simulink model "Simulink_Model"  (R2020b)
settings: Solver=FixedStepAuto  StartTime=0.0  StopTime=12  FixedStep=1  RelTol=1e-3
values from neighbouring files (symbols this model uses):
  ConstantA = Constants{1}    [Load_config.m]
  ConstantB = Constants{2}    [Load_config.m]
  ConstantC = Constants{3}    [Load_config.m]
  ConstantD = Constants{4}    [Load_config.m]
  ConstantE = Constants{5}    [Load_config.m]
  ConstantF = Constants{6}    [Load_config.m]
  ConstantG = Constants{7}    [Load_config.m]
  ConstantH = Constants{8}    [Load_config.m]
  ConstantI = Constants{9}    [Load_config.m]
  ConstantJ = Constants{18}    [Load_config.m]
  ConstantK = Constants{19}    [Load_config.m]
  ConstantL = Constants{20}    [Load_config.m]
  ConstantM = Constants{21}    [Load_config.m]
  ConstantO = Constants{22}    [Load_config.m]
undefined symbols (not defined in the file or in its folder): A1052, A2, F2, G1052, H2, K1052
libraries: simulink x32, sldvlib x22
(part 2 of 3)

== system Simulink_Model/Subsystem/Requirement3/ComputeOutputD[0][0] ==
  OutputB[x][y] : Inport
  Compare To Constant1 : simulink/Logic and Bit Operations/Compare To Constant  relop=>=  const=0  OutDataTypeStr=boolean
  Constant : Constant  Value=0.5
  Constant1 : Constant  Value=ConstantD
  Constant2 : Constant  Value=ConstantB
  Constant3 : Constant  Value=ConstantC
  Constant4 : Constant  Value=ConstantE
  Constant5 : Constant  Value=ConstantI
  Divide : Product  Inputs=*/
  Gain : Gain  Gain=-1
  Product : Product  Inputs=3
  Product1 : Product  Inputs=3
  Product2 : Product
  Sum : Sum  Inputs=|++
  Switch2 : Switch  Criteria=u2 > Threshold
  OutputD[x][y] : Outport
  wires:
  OutputB[x][y]/1 -> Product/3
  Constant1/1 -> Product/1  "ConstantD"
  Constant2/1 -> Product/2  "ConstantB"
  Constant4/1 -> Product1/2  "ConstantE"
  Constant3/1 -> Product1/1  "ConstantC"
  Constant5/1 -> Product1/3  "ConstantI"
  Product/1 -> Sum/1, Compare To Constant1/1
  Gain/1 -> Switch2/3
  Product1/1 -> Divide/2, Product2/2
  Product2/1 -> Switch2/1, Gain/1
  Constant/1 -> Product2/1
  Divide/1 -> OutputD[x][y]/1
  Sum/1 -> Divide/1
  Compare To Constant1/1 -> Switch2/2
  Switch2/1 -> Sum/2

== system Simulink_Model/Subsystem/Requirement3/ComputeOutputD[0][1] ==
  OutputB[x][y] : Inport
  Compare To Constant1 : simulink/Logic and Bit Operations/Compare To Constant  relop=>=  const=0  OutDataTypeStr=boolean
  Constant : Constant  Value=0.5
  Constant1 : Constant  Value=ConstantD
  Constant2 : Constant  Value=ConstantB
  Constant3 : Constant  Value=ConstantC
  Constant4 : Constant  Value=ConstantE
  Constant5 : Constant  Value=ConstantI
  Divide : Product  Inputs=*/
  Gain : Gain  Gain=-1
  Product : Product  Inputs=3
  Product1 : Product  Inputs=3
  Product2 : Product
  Sum : Sum  Inputs=|++
  Switch2 : Switch  Criteria=u2 > Threshold
  OutputD[x][y] : Outport
  wires:
  OutputB[x][y]/1 -> Product/3
  Constant1/1 -> Product/1  "ConstantD"
  Constant2/1 -> Product/2  "ConstantB"
  Constant4/1 -> Product1/2  "ConstantE"
  Constant3/1 -> Product1/1  "ConstantC"
  Constant5/1 -> Product1/3  "ConstantI"
  Product/1 -> Sum/1, Compare To Constant1/1
  Gain/1 -> Switch2/3
  Product1/1 -> Divide/2, Product2/2
  Product2/1 -> Switch2/1, Gain/1
  Constant/1 -> Product2/1
  Divide/1 -> OutputD[x][y]/1
  Sum/1 -> Divide/1
  Compare To Constant1/1 -> Switch2/2
  Switch2/1 -> Sum/2

== system Simulink_Model/Subsystem/Requirement3/ComputeOutputD[1][0] ==
  OutputB[x][y] : Inport
  Compare To Constant1 : simulink/Logic and Bit Operations/Compare To Constant  relop=>=  const=0  OutDataTypeStr=boolean
  Constant : Constant  Value=0.5
  Constant1 : Constant  Value=ConstantD
  Constant2 : Constant  Value=ConstantB
  Constant3 : Constant  Value=ConstantC
  Constant4 : Constant  Value=ConstantE
  Constant5 : Constant  Value=ConstantI
  Divide : Product  Inputs=*/
  Gain : Gain  Gain=-1
  Product : Product  Inputs=3
  Product1 : Product  Inputs=3
  Product2 : Product
  Sum : Sum  Inputs=|++
  Switch2 : Switch  Criteria=u2 > Threshold
  OutputD[x][y] : Outport
  wires:
  OutputB[x][y]/1 -> Product/3
  Constant1/1 -> Product/1  "ConstantD"
  Constant2/1 -> Product/2  "ConstantB"
  Constant4/1 -> Product1/2  "ConstantE"
  Constant3/1 -> Product1/1  "ConstantC"
  Constant5/1 -> Product1/3  "ConstantI"
  Product/1 -> Sum/1, Compare To Constant1/1
  Gain/1 -> Switch2/3
  Product1/1 -> Divide/2, Product2/2
  Product2/1 -> Switch2/1, Gain/1
  Constant/1 -> Product2/1
  Divide/1 -> OutputD[x][y]/1
  Sum/1 -> Divide/1
  Compare To Constant1/1 -> Switch2/2
  Switch2/1 -> Sum/2

== system Simulink_Model/Subsystem/Requirement3/ComputeOutputD[1][1] ==
  OutputB[x][y] : Inport
  Compare To Constant1 : simulink/Logic and Bit Operations/Compare To Constant  relop=>=  const=0  OutDataTypeStr=boolean
  Constant : Constant  Value=0.5
  Constant1 : Constant  Value=ConstantD
  Constant2 : Constant  Value=ConstantB
  Constant3 : Constant  Value=ConstantC
  Constant4 : Constant  Value=ConstantE
  Constant5 : Constant  Value=ConstantI
  Divide : Product  Inputs=*/
  Gain : Gain  Gain=-1
  Product : Product  Inputs=3
  Product1 : Product  Inputs=3
  Product2 : Product
  Sum : Sum  Inputs=|++
  Switch2 : Switch  Criteria=u2 > Threshold
  OutputD[x][y] : Outport
  wires:
  OutputB[x][y]/1 -> Product/3
  Constant1/1 -> Product/1  "ConstantD"
  Constant2/1 -> Product/2  "ConstantB"
  Constant4/1 -> Product1/2  "ConstantE"
  Constant3/1 -> Product1/1  "ConstantC"
  Constant5/1 -> Product1/3  "ConstantI"
  Product/1 -> Sum/1, Compare To Constant1/1
  Gain/1 -> Switch2/3
  Product1/1 -> Divide/2, Product2/2
  Product2/1 -> Switch2/1, Gain/1
  Constant/1 -> Product2/1
  Divide/1 -> OutputD[x][y]/1
  Sum/1 -> Divide/1
  Compare To Constant1/1 -> Switch2/2
  Switch2/1 -> Sum/2

== system Simulink_Model/Subsystem/Requirement4/ComputeOutput[0][0] ==
  OutputB[x][y] : Inport
  OutputD[x][y] : Inport  Port=2
  OutputEOld[x][y] : Inport  Port=3
  OutputFOld[x][y] : Inport  Port=4
  Abs : Abs
  Abs1 : Abs
  Bias : Bias  Bias=50
  Constant : Constant  Value=0
  Constant1 : Constant  Value=0
  Constant2 : Constant  Value=100
  Constant3 : Constant  Value=0
  Constant4 : Constant  Value=ConstantI
  Constant6 : Constant  Value=ConstantC
  Delay : Delay  DelayLength=1  InitialCondition=0
  Delay1 : Delay  DelayLength=1  InitialCondition=0
  Divide : Product  Inputs=*/
  Max : MinMax  Function=max  Inputs=2
  Product : Product
  Product1 : Product
  Relational Operator : RelationalOperator  Operator===  OutDataTypeStr=boolean  RndMeth=Simplest
  Relational Operator1 : RelationalOperator  Operator=>  OutDataTypeStr=boolean  RndMeth=Simplest
  Subtract : Sum  Inputs=+-
  Switch : Switch
  Switch1 : Switch
  Switch2 : Switch
  OutputE[x][y] : Outport
  OutputF[x][y] : Outport  Port=2
  wires:
  Constant/1 -> Relational Operator/1
  OutputB[x][y]/1 -> Relational Operator/2
  Relational Operator/1 -> Switch2/2, Switch/2
  Switch/1 -> Product1/1, OutputE[x][y]/1
  OutputD[x][y]/1 -> Product/1, Switch/3
  Constant1/1 -> Switch1/3, Relational Operator1/1
  OutputFOld[x][y]/1 -> Delay1/1
  Relational Operator1/1 -> Switch1/2
  OutputEOld[x][y]/1 -> Delay/1
  Switch1/1 -> Switch/1
  Switch2/1 -> OutputF[x][y]/1
  Constant4/1 -> Product/2  "ConstantI"
  Product/1 -> Abs/1
  Abs/1 -> Bias/1
  Bias/1 -> Divide/1
  Constant2/1 -> Divide/2
  Divide/1 -> Switch2/1
  Subtract/1 -> Max/1
  Constant3/1 -> Max/2
  Constant6/1 -> Product1/2  "ConstantC"
  Product1/1 -> Abs1/1
  Abs1/1 -> Subtract/2
  Max/1 -> Switch2/3
  Delay/1 -> Switch1/1
  Delay1/1 -> Subtract/1, Relational Operator1/2

== system Simulink_Model/Subsystem/Requirement4/ComputeOutput[0][1] ==
  OutputB[x][y] : Inport
  OutputD[x][y] : Inport  Port=2
  OutputEOld[x][y] : Inport  Port=3
  OutputFOld[x][y] : Inport  Port=4
  Abs : Abs
  Abs1 : Abs
  Bias : Bias  Bias=50
  Constant : Constant  Value=0
  Constant1 : Constant  Value=0
  Constant2 : Constant  Value=100
  Constant3 : Constant  Value=0
  Constant4 : Constant  Value=ConstantI
  Constant6 : Constant  Value=ConstantC
  Delay : Delay  DelayLength=1  InitialCondition=0
  Delay1 : Delay  DelayLength=1  InitialCondition=0
  Divide : Product  Inputs=*/
  Max : MinMax  Function=max  Inputs=2
  Product : Product
  Product1 : Product
  Relational Operator : RelationalOperator  Operator===  OutDataTypeStr=boolean  RndMeth=Simplest
  Relational Operator1 : RelationalOperator  Operator=>  OutDataTypeStr=boolean  RndMeth=Simplest
  Subtract : Sum  Inputs=+-
  Switch : Switch
  Switch1 : Switch
  Switch2 : Switch
  OutputE[x][y] : Outport
  OutputF[x][y] : Outport  Port=2
  wires:
  Constant/1 -> Relational Operator/1
  OutputB[x][y]/1 -> Relational Operator/2
  Relational Operator/1 -> Switch2/2, Switch/2
  Switch/1 -> OutputE[x][y]/1
  OutputD[x][y]/1 -> Product/1, Switch/3
  Constant1/1 -> Switch1/3, Relational Operator1/1
  OutputFOld[x][y]/1 -> Delay1/1
  Relational Operator1/1 -> Switch1/2
  OutputEOld[x][y]/1 -> Delay/1
  Switch1/1 -> Switch/1, Product1/1
  Switch2/1 -> OutputF[x][y]/1
  Constant4/1 -> Product/2  "ConstantI"
  Product/1 -> Abs/1
  Abs/1 -> Bias/1
  Bias/1 -> Divide/1
  Constant2/1 -> Divide/2
  Divide/1 -> Subtract/1, Switch2/1
  Subtract/1 -> Max/1
  Constant3/1 -> Max/2
  Constant6/1 -> Product1/2  "ConstantC"
  Product1/1 -> Abs1/1
  Abs1/1 -> Subtract/2
  Max/1 -> Switch2/3
  Delay/1 -> Switch1/1
  Delay1/1 -> Relational Operator1/2

== system Simulink_Model/Subsystem/Requirement4/ComputeOutput[1][0] ==
  OutputB[x][y] : Inport
  OutputD[x][y] : Inport  Port=2
  OutputEOld[x][y] : Inport  Port=3
  OutputFOld[x][y] : Inport  Port=4
  Abs : Abs
  Abs1 : Abs
  Bias : Bias  Bias=50
  Constant : Constant  Value=0
  Constant1 : Constant  Value=0
  Constant2 : Constant  Value=100
  Constant3 : Constant  Value=0
  Constant4 : Constant  Value=ConstantI
  Constant6 : Constant  Value=ConstantC
  Delay : Delay  DelayLength=1  InitialCondition=0
  Delay1 : Delay  DelayLength=1  InitialCondition=0
  Divide : Product  Inputs=*/
  Max : MinMax  Function=max  Inputs=2
  Product : Product
  Product1 : Product
  Relational Operator : RelationalOperator  Operator===  OutDataTypeStr=boolean  RndMeth=Simplest
  Relational Operator1 : RelationalOperator  Operator=>  OutDataTypeStr=boolean  RndMeth=Simplest
  Subtract : Sum  Inputs=+-
  Switch : Switch
  Switch1 : Switch
  Switch2 : Switch
  OutputE[x][y] : Outport
  OutputF[x][y] : Outport  Port=2
  wires:
  Constant/1 -> Relational Operator/1
  OutputB[x][y]/1 -> Relational Operator/2
  Relational Operator/1 -> Switch2/2, Switch/2
  Switch/1 -> OutputE[x][y]/1
  OutputD[x][y]/1 -> Product/1, Switch/3
  Constant1/1 -> Switch1/3, Relational Operator1/1
  OutputFOld[x][y]/1 -> Delay1/1
  Relational Operator1/1 -> Switch1/2
  OutputEOld[x][y]/1 -> Delay/1
  Switch1/1 -> Switch/1, Product1/1
  Switch2/1 -> OutputF[x][y]/1
  Constant4/1 -> Product/2  "ConstantI"
  Product/1 -> Abs/1
  Abs/1 -> Bias/1
  Bias/1 -> Divide/1
  Constant2/1 -> Divide/2
  Divide/1 -> Subtract/1, Switch2/1
  Subtract/1 -> Max/1
  Constant3/1 -> Max/2
  Constant6/1 -> Product1/2  "ConstantC"
  Product1/1 -> Abs1/1
  Abs1/1 -> Subtract/2
  Max/1 -> Switch2/3
  Delay/1 -> Switch1/1
  Delay1/1 -> Relational Operator1/2

== system Simulink_Model/Subsystem/Requirement4/ComputeOutput[1][1] ==
  OutputB[x][y] : Inport
  OutputD[x][y] : Inport  Port=2
  OutputEOld[x][y] : Inport  Port=3
  OutputFOld[x][y] : Inport  Port=4
  Abs : Abs
  Abs1 : Abs
  Bias : Bias  Bias=50
  Constant : Constant  Value=0
  Constant1 : Constant  Value=0
  Constant2 : Constant  Value=100
  Constant3 : Constant  Value=0
  Constant4 : Constant  Value=ConstantI
  Constant6 : Constant  Value=ConstantC
  Delay : Delay  DelayLength=1  InitialCondition=0
  Delay1 : Delay  DelayLength=1  InitialCondition=0
  Divide : Product  Inputs=*/
  Max : MinMax  Function=max  Inputs=2
  Product : Product
  Product1 : Product
  Relational Operator : RelationalOperator  Operator===  OutDataTypeStr=boolean  RndMeth=Simplest
  Relational Operator1 : RelationalOperator  Operator=>  OutDataTypeStr=boolean  RndMeth=Simplest
  Subtract : Sum  Inputs=+-
  Switch : Switch
  Switch1 : Switch
  Switch2 : Switch
  OutputE[x][y] : Outport
  OutputF[x][y] : Outport  Port=2
  wires:
  Constant/1 -> Relational Operator/1
  OutputB[x][y]/1 -> Relational Operator/2
  Relational Operator/1 -> Switch2/2, Switch/2
  Switch/1 -> OutputE[x][y]/1
  OutputD[x][y]/1 -> Product/1, Switch/3
  Constant1/1 -> Switch1/3, Relational Operator1/1
  OutputFOld[x][y]/1 -> Delay1/1
  Relational Operator1/1 -> Switch1/2
  OutputEOld[x][y]/1 -> Delay/1
  Switch1/1 -> Switch/1, Product1/1
  Switch2/1 -> OutputF[x][y]/1
  Constant4/1 -> Product/2  "ConstantI"
  Product/1 -> Abs/1
  Abs/1 -> Bias/1
  Bias/1 -> Divide/1
  Constant2/1 -> Divide/2
  Divide/1 -> Subtract/1, Switch2/1
  Subtract/1 -> Max/1
  Constant3/1 -> Max/2
  Constant6/1 -> Product1/2  "ConstantC"
  Product1/1 -> Abs1/1
  Abs1/1 -> Subtract/2
  Max/1 -> Switch2/3
  Delay/1 -> Switch1/1
  Delay1/1 -> Relational Operator1/2

== system Simulink_Model/Subsystem/Requirement5/ComputeOutputG[0][0] ==
  OutputB[x][y] : Inport
  SignalB[x] : Inport  Port=2
  SignalC[x][y] : Inport  Port=3
  Compare To Constant1 : simulink/Logic and Bit Operations/Compare To Constant  relop=>=  const=0  OutDataTypeStr=boolean
  Constant : Constant  Value=0.5
  Constant1 : Constant  Value=ConstantD
  Constant2 : Constant  Value=ConstantB
  Constant3 : Constant  Value=ConstantC
  Constant4 : Constant  Value=ConstantE
  Constant5 : Constant  Value=ConstantI
  Divide : Product  Inputs=*/
  Gain : Gain  Gain=-1
  Gain1 : Gain  Gain=2
  Product : Product  Inputs=3
  Product1 : Product  Inputs=3
  Product2 : Product
  Sum : Sum  Inputs=|++
  Sum1 : Sum  Inputs=|+++
  Switch2 : Switch  Criteria=u2 > Threshold
  OutputG[x][y] : Outport
  wires:
  Constant3/1 -> Product1/1  "ConstantC"
  Constant/1 -> Product2/1
  Product/1 -> Sum/1, Compare To Constant1/1
  Sum/1 -> Divide/1
  Product1/1 -> Divide/2, Product2/2
  Constant1/1 -> Product/1  "ConstantD"
  Constant5/1 -> Product1/3  "ConstantI"
  Constant4/1 -> Product1/2  "ConstantE"
  Constant2/1 -> Product/2  "ConstantB"
  Sum1/1 -> Product/3
  Divide/1 -> OutputG[x][y]/1
  SignalB[x]/1 -> Gain1/1
  Gain1/1 -> Sum1/2
  OutputB[x][y]/1 -> Sum1/1
  SignalC[x][y]/1 -> Sum1/3
  Switch2/1 -> Sum/2
  Gain/1 -> Switch2/3
  Product2/1 -> Gain/1, Switch2/1
  Compare To Constant1/1 -> Switch2/2

== system Simulink_Model/Subsystem/Requirement5/ComputeOutputG[0][1] ==
  OutputB[x][y] : Inport
  SignalB[x] : Inport  Port=2
  SignalC[x][y] : Inport  Port=3
  Compare To Constant1 : simulink/Logic and Bit Operations/Compare To Constant  relop=>=  const=0  OutDataTypeStr=boolean
  Constant : Constant  Value=0.5
  Constant1 : Constant  Value=ConstantD
  Constant2 : Constant  Value=ConstantB
  Constant3 : Constant  Value=ConstantC
  Constant4 : Constant  Value=ConstantE
  Constant5 : Constant  Value=ConstantI
  Divide : Product  Inputs=*/
  Gain : Gain  Gain=-1
  Gain1 : Gain  Gain=2
  Product : Product  Inputs=3
  Product1 : Product  Inputs=3
  Product2 : Product
  Sum : Sum  Inputs=|++
  Sum1 : Sum  Inputs=|+++
  Switch2 : Switch  Criteria=u2 > Threshold
  OutputG[x][y] : Outport
  wires:
  Constant3/1 -> Product1/1  "ConstantC"
  Constant/1 -> Product2/1
  Product/1 -> Sum/1, Compare To Constant1/1
  Sum/1 -> Divide/1
  Product1/1 -> Divide/2, Product2/2
  Constant1/1 -> Product/1  "ConstantD"
  Constant5/1 -> Product1/3  "ConstantI"
  Constant4/1 -> Product1/2  "ConstantE"
  Constant2/1 -> Product/2  "ConstantB"
  Sum1/1 -> Product/3
  Divide/1 -> OutputG[x][y]/1
  SignalB[x]/1 -> Gain1/1
  Gain1/1 -> Sum1/2
  OutputB[x][y]/1 -> Sum1/1
  SignalC[x][y]/1 -> Sum1/3
  Switch2/1 -> Sum/2
  Gain/1 -> Switch2/3
  Product2/1 -> Gain/1, Switch2/1
  Compare To Constant1/1 -> Switch2/2

== system Simulink_Model/Subsystem/Requirement5/ComputeOutputG[1][0] ==
  OutputB[x][y] : Inport
  SignalB[x] : Inport  Port=2
  SignalC[x][y] : Inport  Port=3
  Compare To Constant1 : simulink/Logic and Bit Operations/Compare To Constant  relop=>=  const=0  OutDataTypeStr=boolean
  Constant : Constant  Value=0.5
  Constant1 : Constant  Value=ConstantD
  Constant2 : Constant  Value=ConstantB
  Constant3 : Constant  Value=ConstantC
  Constant4 : Constant  Value=ConstantE
  Constant5 : Constant  Value=ConstantI
  Divide : Product  Inputs=*/
  Gain : Gain  Gain=-1
  Gain1 : Gain  Gain=2
  Product : Product  Inputs=3
  Product1 : Product  Inputs=3
  Product2 : Product
  Sum : Sum  Inputs=|++
  Sum1 : Sum  Inputs=|+++
  Switch2 : Switch  Criteria=u2 > Threshold
  OutputG[x][y] : Outport
  wires:
  Constant3/1 -> Product1/1  "ConstantC"
  Constant/1 -> Product2/1
  Product/1 -> Sum/1, Compare To Constant1/1
  Sum/1 -> Divide/1
  Product1/1 -> Divide/2, Product2/2
  Constant1/1 -> Product/1  "ConstantD"
  Constant5/1 -> Product1/3  "ConstantI"
  Constant4/1 -> Product1/2  "ConstantE"
  Constant2/1 -> Product/2  "ConstantB"
  Sum1/1 -> Product/3
  Divide/1 -> OutputG[x][y]/1
  SignalB[x]/1 -> Gain1/1
  Gain1/1 -> Sum1/2
  OutputB[x][y]/1 -> Sum1/1
  SignalC[x][y]/1 -> Sum1/3
  Switch2/1 -> Sum/2
  Gain/1 -> Switch2/3
  Product2/1 -> Gain/1, Switch2/1
  Compare To Constant1/1 -> Switch2/2

== system Simulink_Model/Subsystem/Requirement5/ComputeOutputG[1][1] ==
  OutputB[x][y] : Inport
  SignalB[x] : Inport  Port=2
  SignalC[x][y] : Inport  Port=3
  Compare To Constant1 : simulink/Logic and Bit Operations/Compare To Constant  relop=>=  const=0  OutDataTypeStr=boolean
  Constant : Constant  Value=0.5
  Constant1 : Constant  Value=ConstantD
  Constant2 : Constant  Value=ConstantB
  Constant3 : Constant  Value=ConstantC
  Constant4 : Constant  Value=ConstantE
  Constant5 : Constant  Value=ConstantI
  Divide : Product  Inputs=*/
  Gain : Gain  Gain=-1
  Gain1 : Gain  Gain=2
  Product : Product  Inputs=3
  Product1 : Product  Inputs=3
  Product2 : Product
  Sum : Sum  Inputs=|++
  Sum1 : Sum  Inputs=|+++
  Switch2 : Switch  Criteria=u2 > Threshold
  OutputG[x][y] : Outport
  wires:
  Constant3/1 -> Product1/1  "ConstantC"
  Constant/1 -> Product2/1
  Product/1 -> Sum/1, Compare To Constant1/1
  Sum/1 -> Divide/1
  Product1/1 -> Divide/2, Product2/2
  Constant1/1 -> Product/1  "ConstantD"
  Constant5/1 -> Product1/3  "ConstantI"
  Constant4/1 -> Product1/2  "ConstantE"
  Constant2/1 -> Product/2  "ConstantB"
  Sum1/1 -> Product/3
  Divide/1 -> OutputG[x][y]/1
  SignalB[x]/1 -> Gain1/1
  Gain1/1 -> Sum1/2
  OutputB[x][y]/1 -> Sum1/1
  SignalC[x][y]/1 -> Sum1/3
  Switch2/1 -> Sum/2
  Gain/1 -> Switch2/3
  Product2/1 -> Gain/1, Switch2/1
  Compare To Constant1/1 -> Switch2/2

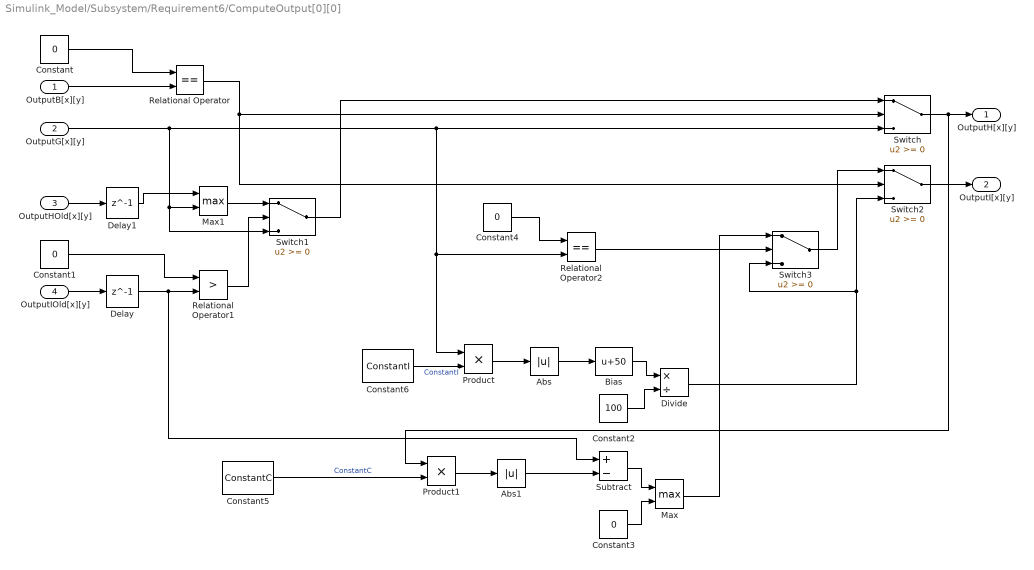
== system Simulink_Model/Subsystem/Requirement6/ComputeOutput[0][0] ==
  OutputB[x][y] : Inport
  OutputG[x][y] : Inport  Port=2
  OutputHOld[x][y] : Inport  Port=3
  OutputIOld[x][y] : Inport  Port=4
  Abs : Abs
  Abs1 : Abs
  Bias : Bias  Bias=50
  Constant{,1,3..4} (4 alike) : Constant  Value=0
  Constant2 : Constant  Value=100
  Constant5 : Constant  Value=ConstantC
  Constant6 : Constant  Value=ConstantI
  Delay : Delay  DelayLength=1  InitialCondition=0
  Delay1 : Delay  DelayLength=1  InitialCondition=0
  Divide : Product  Inputs=*/
  Max : MinMax  Function=max  Inputs=2
  Max1 : MinMax  Function=max  Inputs=2
  Product : Product
  Product1 : Product
  Relational Operator : RelationalOperator  Operator===  OutDataTypeStr=boolean  RndMeth=Simplest
  Relational Operator1 : RelationalOperator  Operator=>  OutDataTypeStr=boolean  RndMeth=Simplest
  Relational Operator2 : RelationalOperator  Operator===  OutDataTypeStr=boolean  RndMeth=Simplest
  Subtract : Sum  Inputs=+-
  Switch{,1..3} (4 alike) : Switch
  OutputH[x][y] : Outport
  OutputI[x][y] : Outport  Port=2
  wires:
  Constant/1 -> Relational Operator/1
  OutputB[x][y]/1 -> Relational Operator/2
  Relational Operator/1 -> Switch2/2, Switch/2
  Switch/1 -> Product1/1, OutputH[x][y]/1
  OutputG[x][y]/1 -> Relational Operator2/2, Product/1, Switch/3, Switch1/3, Max1/2
  Constant1/1 -> Relational Operator1/1
  OutputIOld[x][y]/1 -> Delay/1
  Relational Operator1/1 -> Switch1/2
  OutputHOld[x][y]/1 -> Delay1/1
  Switch1/1 -> Switch/1
  Switch2/1 -> OutputI[x][y]/1
  Constant6/1 -> Product/2  "ConstantI"
  Product/1 -> Abs/1
  Abs/1 -> Bias/1
  Bias/1 -> Divide/1
  Constant2/1 -> Divide/2
  Subtract/1 -> Max/1
  Constant3/1 -> Max/2
  Constant5/1 -> Product1/2  "ConstantC"
  Product1/1 -> Abs1/1
  Abs1/1 -> Subtract/2
  Constant4/1 -> Relational Operator2/1
  Relational Operator2/1 -> Switch3/2
  Switch3/1 -> Switch2/1
  Divide/1 -> Switch3/3, Switch2/3
  Max/1 -> Switch3/1
  Delay/1 -> Subtract/1, Relational Operator1/2
  Max1/1 -> Switch1/1
  Delay1/1 -> Max1/1

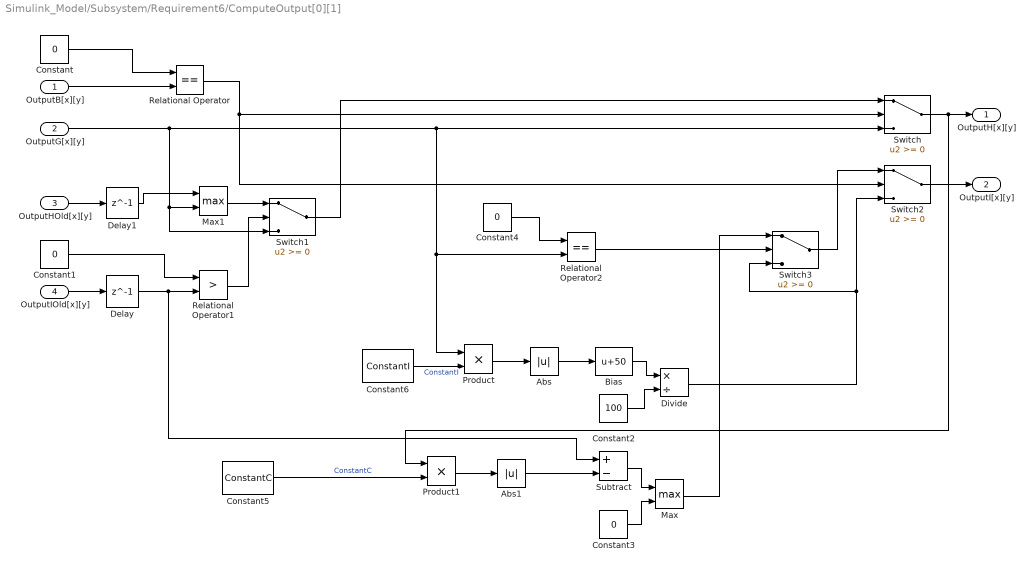
== system Simulink_Model/Subsystem/Requirement6/ComputeOutput[0][1] ==
  OutputB[x][y] : Inport
  OutputG[x][y] : Inport  Port=2
  OutputHOld[x][y] : Inport  Port=3
  OutputIOld[x][y] : Inport  Port=4
  Abs : Abs
  Abs1 : Abs
  Bias : Bias  Bias=50
  Constant{,1,3..4} (4 alike) : Constant  Value=0
  Constant2 : Constant  Value=100
  Constant5 : Constant  Value=ConstantC
  Constant6 : Constant  Value=ConstantI
  Delay : Delay  DelayLength=1  InitialCondition=0
  Delay1 : Delay  DelayLength=1  InitialCondition=0
  Divide : Product  Inputs=*/
  Max : MinMax  Function=max  Inputs=2
  Max1 : MinMax  Function=max  Inputs=2
  Product : Product
  Product1 : Product
  Relational Operator : RelationalOperator  Operator===  OutDataTypeStr=boolean  RndMeth=Simplest
  Relational Operator1 : RelationalOperator  Operator=>  OutDataTypeStr=boolean  RndMeth=Simplest
  Relational Operator2 : RelationalOperator  Operator===  OutDataTypeStr=boolean  RndMeth=Simplest
  Subtract : Sum  Inputs=+-
  Switch{,1..3} (4 alike) : Switch
  OutputH[x][y] : Outport
  OutputI[x][y] : Outport  Port=2
  wires:
  Constant/1 -> Relational Operator/1
  OutputB[x][y]/1 -> Relational Operator/2
  Relational Operator/1 -> Switch2/2, Switch/2
  Switch/1 -> Product1/1, OutputH[x][y]/1
  OutputG[x][y]/1 -> Relational Operator2/2, Product/1, Switch/3, Switch1/3, Max1/2
  Constant1/1 -> Relational Operator1/1
  OutputIOld[x][y]/1 -> Delay/1
  Relational Operator1/1 -> Switch1/2
  OutputHOld[x][y]/1 -> Delay1/1
  Switch1/1 -> Switch/1
  Switch2/1 -> OutputI[x][y]/1
  Constant6/1 -> Product/2  "ConstantI"
  Product/1 -> Abs/1
  Abs/1 -> Bias/1
  Bias/1 -> Divide/1
  Constant2/1 -> Divide/2
  Subtract/1 -> Max/1
  Constant3/1 -> Max/2
  Constant5/1 -> Product1/2  "ConstantC"
  Product1/1 -> Abs1/1
  Abs1/1 -> Subtract/2
  Constant4/1 -> Relational Operator2/1
  Relational Operator2/1 -> Switch3/2
  Switch3/1 -> Switch2/1
  Divide/1 -> Switch3/3, Switch2/3
  Max/1 -> Switch3/1
  Delay/1 -> Subtract/1, Relational Operator1/2
  Max1/1 -> Switch1/1
  Delay1/1 -> Max1/1

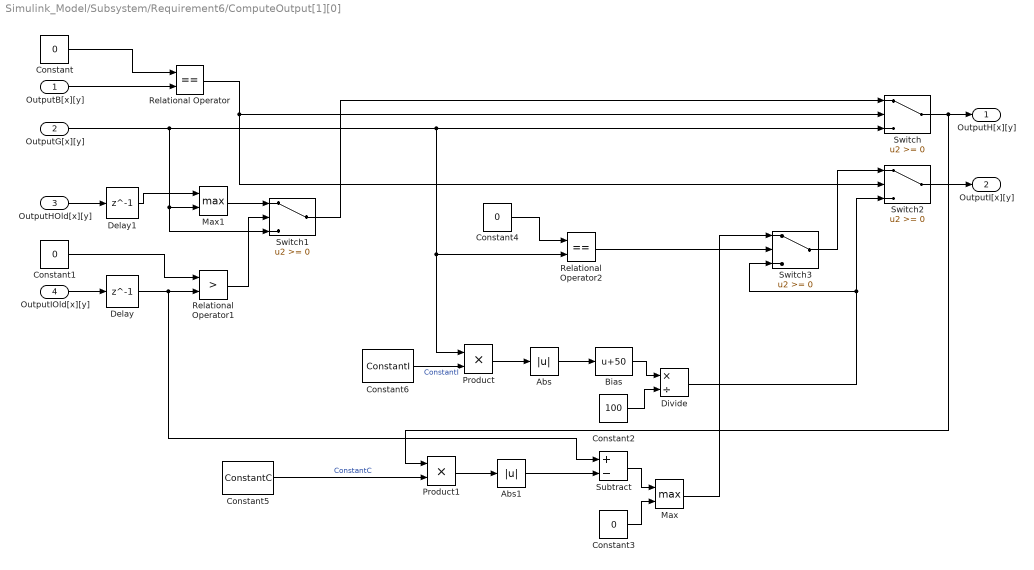
== system Simulink_Model/Subsystem/Requirement6/ComputeOutput[1][0] ==
  OutputB[x][y] : Inport
  OutputG[x][y] : Inport  Port=2
  OutputHOld[x][y] : Inport  Port=3
  OutputIOld[x][y] : Inport  Port=4
  Abs : Abs
  Abs1 : Abs
  Bias : Bias  Bias=50
  Constant{,1,3..4} (4 alike) : Constant  Value=0
  Constant2 : Constant  Value=100
  Constant5 : Constant  Value=ConstantC
  Constant6 : Constant  Value=ConstantI
  Delay : Delay  DelayLength=1  InitialCondition=0
  Delay1 : Delay  DelayLength=1  InitialCondition=0
  Divide : Product  Inputs=*/
  Max : MinMax  Function=max  Inputs=2
  Max1 : MinMax  Function=max  Inputs=2
  Product : Product
  Product1 : Product
  Relational Operator : RelationalOperator  Operator===  OutDataTypeStr=boolean  RndMeth=Simplest
  Relational Operator1 : RelationalOperator  Operator=>  OutDataTypeStr=boolean  RndMeth=Simplest
  Relational Operator2 : RelationalOperator  Operator===  OutDataTypeStr=boolean  RndMeth=Simplest
  Subtract : Sum  Inputs=+-
  Switch{,1..3} (4 alike) : Switch
  OutputH[x][y] : Outport
  OutputI[x][y] : Outport  Port=2
  wires:
  Constant/1 -> Relational Operator/1
  OutputB[x][y]/1 -> Relational Operator/2
  Relational Operator/1 -> Switch2/2, Switch/2
  Switch/1 -> Product1/1, OutputH[x][y]/1
  OutputG[x][y]/1 -> Relational Operator2/2, Product/1, Switch/3, Switch1/3, Max1/2
  Constant1/1 -> Relational Operator1/1
  OutputIOld[x][y]/1 -> Delay/1
  Relational Operator1/1 -> Switch1/2
  OutputHOld[x][y]/1 -> Delay1/1
  Switch1/1 -> Switch/1
  Switch2/1 -> OutputI[x][y]/1
  Constant6/1 -> Product/2  "ConstantI"
  Product/1 -> Abs/1
  Abs/1 -> Bias/1
  Bias/1 -> Divide/1
  Constant2/1 -> Divide/2
  Subtract/1 -> Max/1
  Constant3/1 -> Max/2
  Constant5/1 -> Product1/2  "ConstantC"
  Product1/1 -> Abs1/1
  Abs1/1 -> Subtract/2
  Constant4/1 -> Relational Operator2/1
  Relational Operator2/1 -> Switch3/2
  Switch3/1 -> Switch2/1
  Divide/1 -> Switch3/3, Switch2/3
  Max/1 -> Switch3/1
  Delay/1 -> Subtract/1, Relational Operator1/2
  Max1/1 -> Switch1/1
  Delay1/1 -> Max1/1

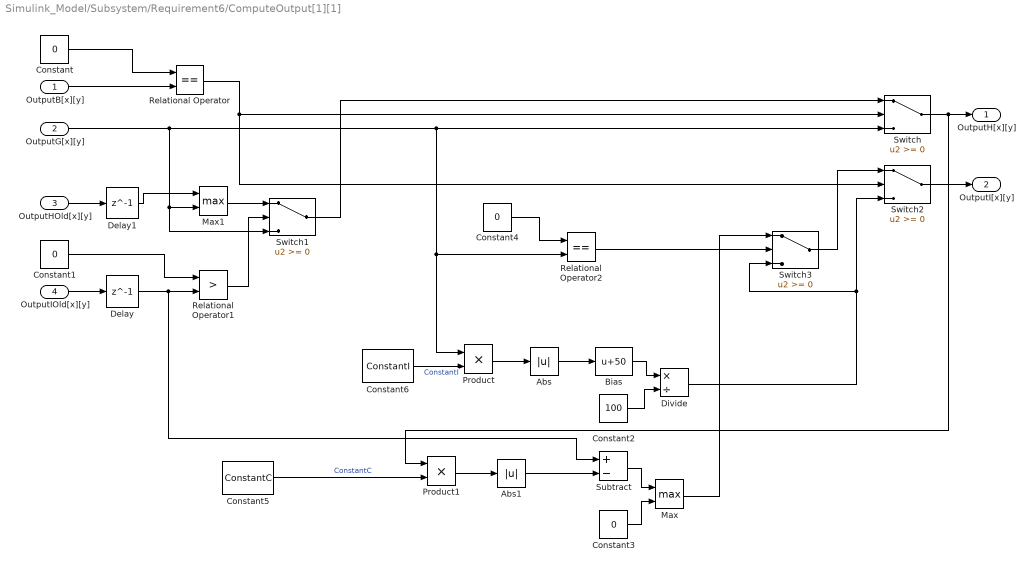
== system Simulink_Model/Subsystem/Requirement6/ComputeOutput[1][1] ==
  OutputB[x][y] : Inport
  OutputG[x][y] : Inport  Port=2
  OutputHOld[x][y] : Inport  Port=3
  OutputIOld[x][y] : Inport  Port=4
  Abs : Abs
  Abs1 : Abs
  Bias : Bias  Bias=50
  Constant{,1,3..4} (4 alike) : Constant  Value=0
  Constant2 : Constant  Value=100
  Constant5 : Constant  Value=ConstantC
  Constant6 : Constant  Value=ConstantI
  Delay : Delay  DelayLength=1  InitialCondition=0
  Delay1 : Delay  DelayLength=1  InitialCondition=0
  Divide : Product  Inputs=*/
  Max : MinMax  Function=max  Inputs=2
  Max1 : MinMax  Function=max  Inputs=2
  Product : Product
  Product1 : Product
  Relational Operator : RelationalOperator  Operator===  OutDataTypeStr=boolean  RndMeth=Simplest
  Relational Operator1 : RelationalOperator  Operator=>  OutDataTypeStr=boolean  RndMeth=Simplest
  Relational Operator2 : RelationalOperator  Operator===  OutDataTypeStr=boolean  RndMeth=Simplest
  Subtract : Sum  Inputs=+-
  Switch{,1..3} (4 alike) : Switch
  OutputH[x][y] : Outport
  OutputI[x][y] : Outport  Port=2
  wires:
  Constant/1 -> Relational Operator/1
  OutputB[x][y]/1 -> Relational Operator/2
  Relational Operator/1 -> Switch2/2, Switch/2
  Switch/1 -> Product1/1, OutputH[x][y]/1
  OutputG[x][y]/1 -> Relational Operator2/2, Product/1, Switch/3, Switch1/3, Max1/2
  Constant1/1 -> Relational Operator1/1
  OutputIOld[x][y]/1 -> Delay/1
  Relational Operator1/1 -> Switch1/2
  OutputHOld[x][y]/1 -> Delay1/1
  Switch1/1 -> Switch/1
  Switch2/1 -> OutputI[x][y]/1
  Constant6/1 -> Product/2  "ConstantI"
  Product/1 -> Abs/1
  Abs/1 -> Bias/1
  Bias/1 -> Divide/1
  Constant2/1 -> Divide/2
  Subtract/1 -> Max/1
  Constant3/1 -> Max/2
  Constant5/1 -> Product1/2  "ConstantC"
  Product1/1 -> Abs1/1
  Abs1/1 -> Subtract/2
  Constant4/1 -> Relational Operator2/1
  Relational Operator2/1 -> Switch3/2
  Switch3/1 -> Switch2/1
  Divide/1 -> Switch3/3, Switch2/3
  Max/1 -> Switch3/1
  Delay/1 -> Subtract/1, Relational Operator1/2
  Max1/1 -> Switch1/1
  Delay1/1 -> Max1/1

== system Simulink_Model/Subsystem/Requirement7/ComputeOutputJ[0][0] ==
  OutputB[x][y] : Inport
  SignalB[x] : Inport  Port=2
  SignalC[x][y] : Inport  Port=3
  Compare To Constant1 : simulink/Logic and Bit Operations/Compare To Constant  relop=>=  const=0  OutDataTypeStr=boolean
  Constant : Constant  Value=0.5
  Constant1 : Constant  Value=ConstantD
  Constant2 : Constant  Value=ConstantB
  Constant3 : Constant  Value=ConstantC
  Constant4 : Constant  Value=ConstantE
  Constant5 : Constant  Value=ConstantI
  Divide : Product  Inputs=*/
  Gain : Gain  Gain=-1
  Gain1 : Gain  Gain=2
  Product : Product  Inputs=3
  Product1 : Product  Inputs=3
  Product2 : Product
  Scope : Scope
  Sum : Sum  Inputs=|++
  Sum1 : Sum  Inputs=|+--
  Switch2 : Switch  Criteria=u2 > Threshold
  OutputJ[x][y] : Outport
  wires:
  Constant3/1 -> Product1/1  "ConstantC"
  Constant/1 -> Product2/1
  Sum/1 -> Divide/1
  Product1/1 -> Divide/2, Product2/2
  Constant1/1 -> Product/1  "ConstantD"
  Constant5/1 -> Product1/3  "ConstantI"
  Constant4/1 -> Product1/2  "ConstantE"
  Constant2/1 -> Product/2  "ConstantB"
  Sum1/1 -> Product/3
  Divide/1 -> OutputJ[x][y]/1
  SignalB[x]/1 -> Gain1/1
  Gain1/1 -> Sum1/2
  OutputB[x][y]/1 -> Sum1/1
  SignalC[x][y]/1 -> Sum1/3
  Switch2/1 -> Sum/2
  Product/1 -> Scope/1, Compare To Constant1/1, Sum/1
  Gain/1 -> Switch2/3
  Product2/1 -> Switch2/1, Gain/1
  Compare To Constant1/1 -> Switch2/2

== system Simulink_Model/Subsystem/Requirement7/ComputeOutputJ[0][1] ==
  OutputB[x][y] : Inport
  SignalB[x] : Inport  Port=2
  SignalC[x][y] : Inport  Port=3
  Compare To Constant1 : simulink/Logic and Bit Operations/Compare To Constant  relop=>=  const=0  OutDataTypeStr=boolean
  Constant : Constant  Value=0.5
  Constant1 : Constant  Value=ConstantD
  Constant2 : Constant  Value=ConstantB
  Constant3 : Constant  Value=ConstantC
  Constant4 : Constant  Value=ConstantE
  Constant5 : Constant  Value=ConstantI
  Divide : Product  Inputs=*/
  Gain : Gain  Gain=-1
  Gain1 : Gain  Gain=2
  Product : Product  Inputs=3
  Product1 : Product  Inputs=3
  Product2 : Product
  Sum : Sum  Inputs=|++
  Sum1 : Sum  Inputs=|+--
  Switch2 : Switch  Criteria=u2 > Threshold
  OutputJ[x][y] : Outport
  wires:
  Constant3/1 -> Product1/1  "ConstantC"
  Constant/1 -> Product2/1
  Sum/1 -> Divide/1
  Product1/1 -> Divide/2, Product2/2
  Constant1/1 -> Product/1  "ConstantD"
  Constant5/1 -> Product1/3  "ConstantI"
  Constant4/1 -> Product1/2  "ConstantE"
  Constant2/1 -> Product/2  "ConstantB"
  Sum1/1 -> Product/3
  Divide/1 -> OutputJ[x][y]/1
  SignalB[x]/1 -> Gain1/1
  Gain1/1 -> Sum1/2
  OutputB[x][y]/1 -> Sum1/1
  SignalC[x][y]/1 -> Sum1/3
  Switch2/1 -> Sum/2
  Product/1 -> Compare To Constant1/1, Sum/1
  Gain/1 -> Switch2/3
  Product2/1 -> Switch2/1, Gain/1
  Compare To Constant1/1 -> Switch2/2

== system Simulink_Model/Subsystem/Requirement7/ComputeOutputJ[1][0] ==
  OutputB[x][y] : Inport
  SignalB[x] : Inport  Port=2
  SignalC[x][y] : Inport  Port=3
  Compare To Constant1 : simulink/Logic and Bit Operations/Compare To Constant  relop=>=  const=0  OutDataTypeStr=boolean
  Constant : Constant  Value=0.5
  Constant1 : Constant  Value=ConstantD
  Constant2 : Constant  Value=ConstantB
  Constant3 : Constant  Value=ConstantC
  Constant4 : Constant  Value=ConstantE
  Constant5 : Constant  Value=ConstantI
  Divide : Product  Inputs=*/
  Gain : Gain  Gain=-1
  Gain1 : Gain  Gain=2
  Product : Product  Inputs=3
  Product1 : Product  Inputs=3
  Product2 : Product
  Sum : Sum  Inputs=|++
  Sum1 : Sum  Inputs=|+--
  Switch2 : Switch  Criteria=u2 > Threshold
  OutputJ[x][y] : Outport
  wires:
  Constant3/1 -> Product1/1  "ConstantC"
  Constant/1 -> Product2/1
  Sum/1 -> Divide/1
  Product1/1 -> Divide/2, Product2/2
  Constant1/1 -> Product/1  "ConstantD"
  Constant5/1 -> Product1/3  "ConstantI"
  Constant4/1 -> Product1/2  "ConstantE"
  Constant2/1 -> Product/2  "ConstantB"
  Sum1/1 -> Product/3
  Divide/1 -> OutputJ[x][y]/1
  SignalB[x]/1 -> Gain1/1
  Gain1/1 -> Sum1/2
  OutputB[x][y]/1 -> Sum1/1
  SignalC[x][y]/1 -> Sum1/3
  Switch2/1 -> Sum/2
  Product/1 -> Compare To Constant1/1, Sum/1
  Gain/1 -> Switch2/3
  Product2/1 -> Switch2/1, Gain/1
  Compare To Constant1/1 -> Switch2/2

== system Simulink_Model/Subsystem/Requirement7/ComputeOutputJ[1][1] ==
  OutputB[x][y] : Inport
  SignalB[x] : Inport  Port=2
  SignalC[x][y] : Inport  Port=3
  Compare To Constant1 : simulink/Logic and Bit Operations/Compare To Constant  relop=>=  const=0  OutDataTypeStr=boolean
  Constant : Constant  Value=0.5
  Constant1 : Constant  Value=ConstantD
  Constant2 : Constant  Value=ConstantB
  Constant3 : Constant  Value=ConstantC
  Constant4 : Constant  Value=ConstantE
  Constant5 : Constant  Value=ConstantI
  Divide : Product  Inputs=*/
  Gain : Gain  Gain=-1
  Gain1 : Gain  Gain=2
  Product : Product  Inputs=3
  Product1 : Product  Inputs=3
  Product2 : Product
  Sum : Sum  Inputs=|++
  Sum1 : Sum  Inputs=|+--
  Switch2 : Switch  Criteria=u2 > Threshold
  OutputJ[x][y] : Outport
  wires:
  Constant3/1 -> Product1/1  "ConstantC"
  Constant/1 -> Product2/1
  Sum/1 -> Divide/1
  Product1/1 -> Divide/2, Product2/2
  Constant1/1 -> Product/1  "ConstantD"
  Constant5/1 -> Product1/3  "ConstantI"
  Constant4/1 -> Product1/2  "ConstantE"
  Constant2/1 -> Product/2  "ConstantB"
  Sum1/1 -> Product/3
  Divide/1 -> OutputJ[x][y]/1
  SignalB[x]/1 -> Gain1/1
  Gain1/1 -> Sum1/2
  OutputB[x][y]/1 -> Sum1/1
  SignalC[x][y]/1 -> Sum1/3
  Switch2/1 -> Sum/2
  Product/1 -> Compare To Constant1/1, Sum/1
  Gain/1 -> Switch2/3
  Product2/1 -> Switch2/1, Gain/1
  Compare To Constant1/1 -> Switch2/2

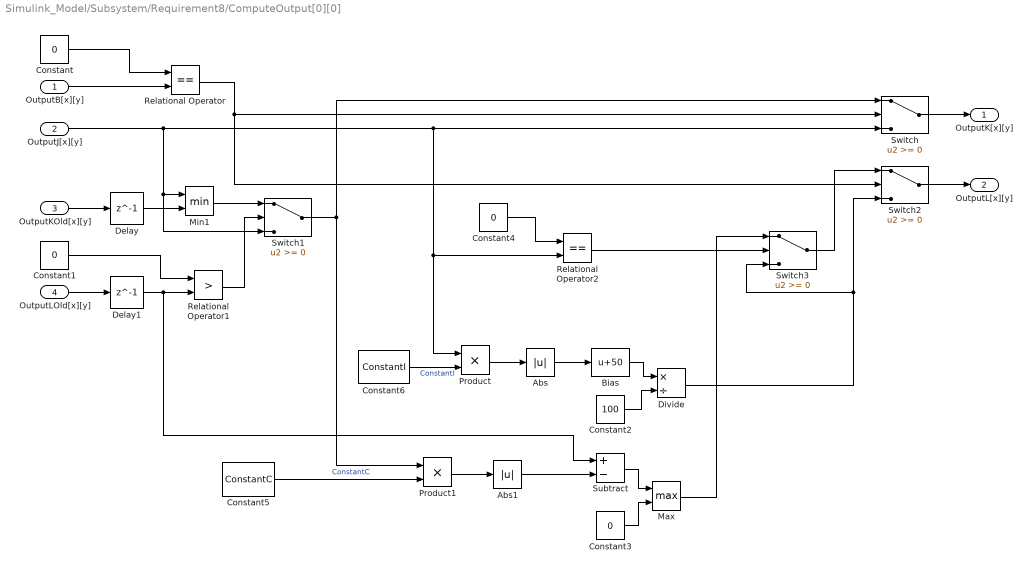
== system Simulink_Model/Subsystem/Requirement8/ComputeOutput[0][0] ==
  OutputB[x][y] : Inport
  OutputJ[x][y] : Inport  Port=2
  OutputKOld[x][y] : Inport  Port=3
  OutputLOld[x][y] : Inport  Port=4
  Abs : Abs
  Abs1 : Abs
  Bias : Bias  Bias=50
  Constant{,1,3..4} (4 alike) : Constant  Value=0
  Constant2 : Constant  Value=100
  Constant5 : Constant  Value=ConstantC
  Constant6 : Constant  Value=ConstantI
  Delay : Delay  DelayLength=1  InitialCondition=0
  Delay1 : Delay  DelayLength=1  InitialCondition=0
  Divide : Product  Inputs=*/
  Max : MinMax  Function=max  Inputs=2
  Min1 : MinMax  Inputs=2
  Product : Product
  Product1 : Product
  Relational Operator : RelationalOperator  Operator===  OutDataTypeStr=boolean  RndMeth=Simplest
  Relational Operator1 : RelationalOperator  Operator=>  OutDataTypeStr=boolean  RndMeth=Simplest
  Relational Operator2 : RelationalOperator  Operator===  OutDataTypeStr=boolean  RndMeth=Simplest
  Subtract : Sum  Inputs=+-
  Switch{,1..3} (4 alike) : Switch
  OutputK[x][y] : Outport
  OutputL[x][y] : Outport  Port=2
  wires:
  Constant/1 -> Relational Operator/1
  OutputB[x][y]/1 -> Relational Operator/2
  Relational Operator/1 -> Switch2/2, Switch/2
  Switch/1 -> OutputK[x][y]/1
  OutputJ[x][y]/1 -> Switch1/3, Min1/1, Relational Operator2/2, Product/1, Switch/3
  Constant1/1 -> Relational Operator1/1
  Relational Operator1/1 -> Switch1/2
  Switch1/1 -> Switch/1, Product1/1
  Switch2/1 -> OutputL[x][y]/1
  Constant6/1 -> Product/2  "ConstantI"
  Product/1 -> Abs/1
  Abs/1 -> Bias/1
  Bias/1 -> Divide/1
  Constant2/1 -> Divide/2
  Subtract/1 -> Max/1
  Constant3/1 -> Max/2
  Constant5/1 -> Product1/2  "ConstantC"
  Product1/1 -> Abs1/1
  Abs1/1 -> Subtract/2
  Constant4/1 -> Relational Operator2/1
  Relational Operator2/1 -> Switch3/2
  Switch3/1 -> Switch2/1
  Divide/1 -> Switch3/3, Switch2/3
  Max/1 -> Switch3/1
  OutputKOld[x][y]/1 -> Delay/1
  OutputLOld[x][y]/1 -> Delay1/1
  Delay1/1 -> Subtract/1, Relational Operator1/2
  Min1/1 -> Switch1/1
  Delay/1 -> Min1/2

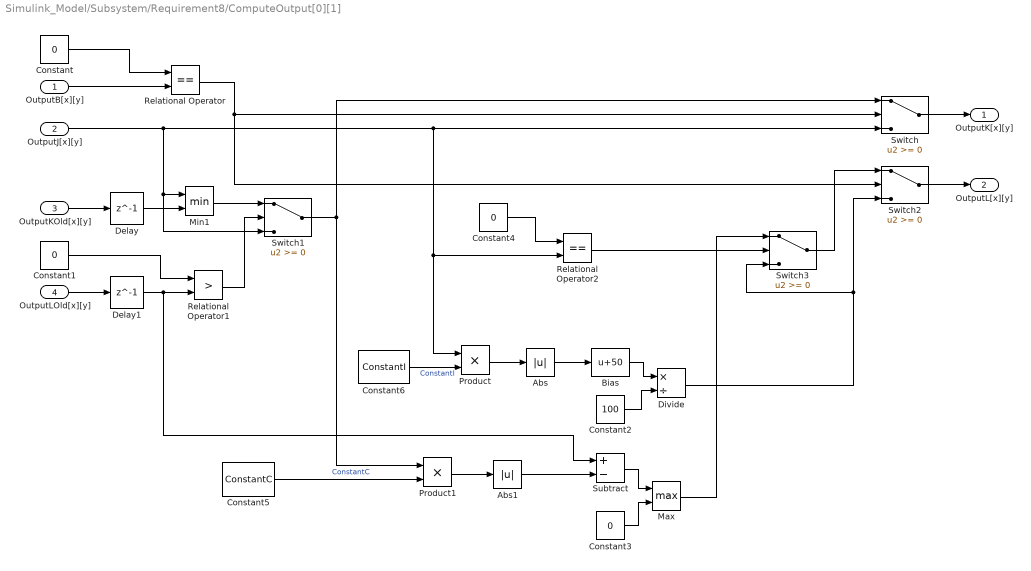
== system Simulink_Model/Subsystem/Requirement8/ComputeOutput[0][1] ==
  OutputB[x][y] : Inport
  OutputJ[x][y] : Inport  Port=2
  OutputKOld[x][y] : Inport  Port=3
  OutputLOld[x][y] : Inport  Port=4
  Abs : Abs
  Abs1 : Abs
  Bias : Bias  Bias=50
  Constant{,1,3..4} (4 alike) : Constant  Value=0
  Constant2 : Constant  Value=100
  Constant5 : Constant  Value=ConstantC
  Constant6 : Constant  Value=ConstantI
  Delay : Delay  DelayLength=1  InitialCondition=0
  Delay1 : Delay  DelayLength=1  InitialCondition=0
  Divide : Product  Inputs=*/
  Max : MinMax  Function=max  Inputs=2
  Min1 : MinMax  Inputs=2
  Product : Product
  Product1 : Product
  Relational Operator : RelationalOperator  Operator===  OutDataTypeStr=boolean  RndMeth=Simplest
  Relational Operator1 : RelationalOperator  Operator=>  OutDataTypeStr=boolean  RndMeth=Simplest
  Relational Operator2 : RelationalOperator  Operator===  OutDataTypeStr=boolean  RndMeth=Simplest
  Subtract : Sum  Inputs=+-
  Switch{,1..3} (4 alike) : Switch
  OutputK[x][y] : Outport
  OutputL[x][y] : Outport  Port=2
  wires:
  Constant/1 -> Relational Operator/1
  OutputB[x][y]/1 -> Relational Operator/2
  Relational Operator/1 -> Switch2/2, Switch/2
  Switch/1 -> OutputK[x][y]/1
  OutputJ[x][y]/1 -> Switch1/3, Min1/1, Relational Operator2/2, Product/1, Switch/3
  Constant1/1 -> Relational Operator1/1
  Relational Operator1/1 -> Switch1/2
  Switch1/1 -> Switch/1, Product1/1
  Switch2/1 -> OutputL[x][y]/1
  Constant6/1 -> Product/2  "ConstantI"
  Product/1 -> Abs/1
  Abs/1 -> Bias/1
  Bias/1 -> Divide/1
  Constant2/1 -> Divide/2
  Subtract/1 -> Max/1
  Constant3/1 -> Max/2
  Constant5/1 -> Product1/2  "ConstantC"
  Product1/1 -> Abs1/1
  Abs1/1 -> Subtract/2
  Constant4/1 -> Relational Operator2/1
  Relational Operator2/1 -> Switch3/2
  Switch3/1 -> Switch2/1
  Divide/1 -> Switch3/3, Switch2/3
  Max/1 -> Switch3/1
  OutputKOld[x][y]/1 -> Delay/1
  OutputLOld[x][y]/1 -> Delay1/1
  Delay1/1 -> Subtract/1, Relational Operator1/2
  Min1/1 -> Switch1/1
  Delay/1 -> Min1/2

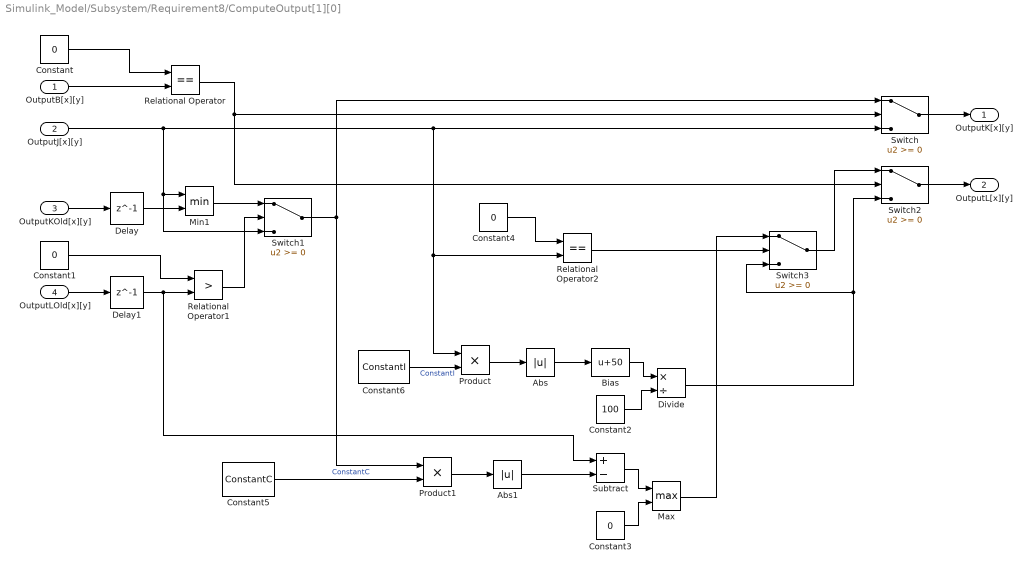
== system Simulink_Model/Subsystem/Requirement8/ComputeOutput[1][0] ==
  OutputB[x][y] : Inport
  OutputJ[x][y] : Inport  Port=2
  OutputKOld[x][y] : Inport  Port=3
  OutputLOld[x][y] : Inport  Port=4
  Abs : Abs
  Abs1 : Abs
  Bias : Bias  Bias=50
  Constant{,1,3..4} (4 alike) : Constant  Value=0
  Constant2 : Constant  Value=100
  Constant5 : Constant  Value=ConstantC
  Constant6 : Constant  Value=ConstantI
  Delay : Delay  DelayLength=1  InitialCondition=0
  Delay1 : Delay  DelayLength=1  InitialCondition=0
  Divide : Product  Inputs=*/
  Max : MinMax  Function=max  Inputs=2
  Min1 : MinMax  Inputs=2
  Product : Product
  Product1 : Product
  Relational Operator : RelationalOperator  Operator===  OutDataTypeStr=boolean  RndMeth=Simplest
  Relational Operator1 : RelationalOperator  Operator=>  OutDataTypeStr=boolean  RndMeth=Simplest
  Relational Operator2 : RelationalOperator  Operator===  OutDataTypeStr=boolean  RndMeth=Simplest
  Subtract : Sum  Inputs=+-
  Switch{,1..3} (4 alike) : Switch
  OutputK[x][y] : Outport
  OutputL[x][y] : Outport  Port=2
  wires:
  Constant/1 -> Relational Operator/1
  OutputB[x][y]/1 -> Relational Operator/2
  Relational Operator/1 -> Switch2/2, Switch/2
  Switch/1 -> OutputK[x][y]/1
  OutputJ[x][y]/1 -> Switch1/3, Min1/1, Relational Operator2/2, Product/1, Switch/3
  Constant1/1 -> Relational Operator1/1
  Relational Operator1/1 -> Switch1/2
  Switch1/1 -> Switch/1, Product1/1
  Switch2/1 -> OutputL[x][y]/1
  Constant6/1 -> Product/2  "ConstantI"
  Product/1 -> Abs/1
  Abs/1 -> Bias/1
  Bias/1 -> Divide/1
  Constant2/1 -> Divide/2
  Subtract/1 -> Max/1
  Constant3/1 -> Max/2
  Constant5/1 -> Product1/2  "ConstantC"
  Product1/1 -> Abs1/1
  Abs1/1 -> Subtract/2
  Constant4/1 -> Relational Operator2/1
  Relational Operator2/1 -> Switch3/2
  Switch3/1 -> Switch2/1
  Divide/1 -> Switch3/3, Switch2/3
  Max/1 -> Switch3/1
  OutputKOld[x][y]/1 -> Delay/1
  OutputLOld[x][y]/1 -> Delay1/1
  Delay1/1 -> Subtract/1, Relational Operator1/2
  Min1/1 -> Switch1/1
  Delay/1 -> Min1/2

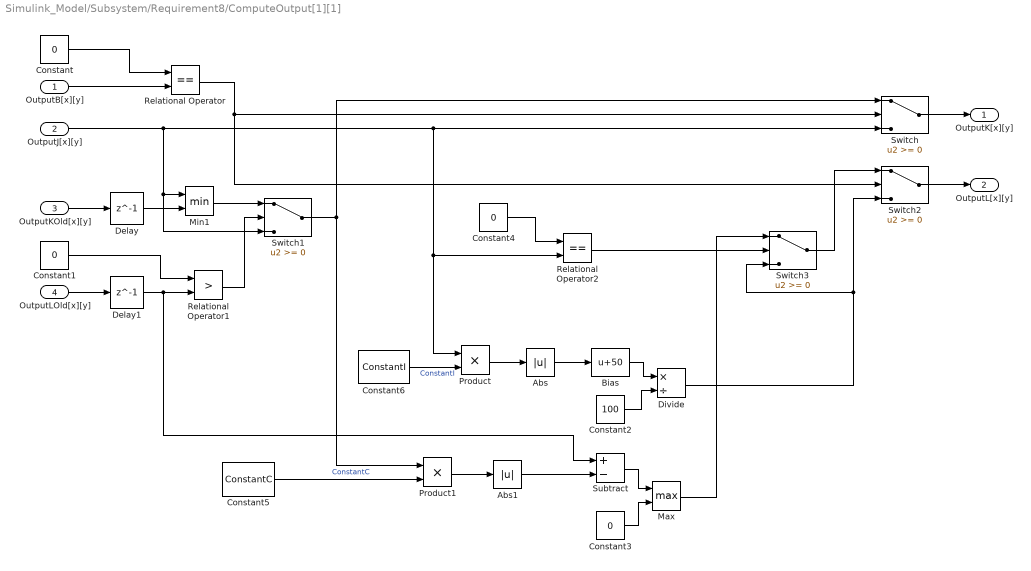
== system Simulink_Model/Subsystem/Requirement8/ComputeOutput[1][1] ==
  OutputB[x][y] : Inport
  OutputJ[x][y] : Inport  Port=2
  OutputKOld[x][y] : Inport  Port=3
  OutputLOld[x][y] : Inport  Port=4
  Abs : Abs
  Abs1 : Abs
  Bias : Bias  Bias=50
  Constant{,1,3..4} (4 alike) : Constant  Value=0
  Constant2 : Constant  Value=100
  Constant5 : Constant  Value=ConstantC
  Constant6 : Constant  Value=ConstantI
  Delay : Delay  DelayLength=1  InitialCondition=0
  Delay1 : Delay  DelayLength=1  InitialCondition=0
  Divide : Product  Inputs=*/
  Max : MinMax  Function=max  Inputs=2
  Min1 : MinMax  Inputs=2
  Product : Product
  Product1 : Product
  Relational Operator : RelationalOperator  Operator===  OutDataTypeStr=boolean  RndMeth=Simplest
  Relational Operator1 : RelationalOperator  Operator=>  OutDataTypeStr=boolean  RndMeth=Simplest
  Relational Operator2 : RelationalOperator  Operator===  OutDataTypeStr=boolean  RndMeth=Simplest
  Subtract : Sum  Inputs=+-
  Switch{,1..3} (4 alike) : Switch
  OutputK[x][y] : Outport
  OutputL[x][y] : Outport  Port=2
  wires:
  Constant/1 -> Relational Operator/1
  OutputB[x][y]/1 -> Relational Operator/2
  Relational Operator/1 -> Switch2/2, Switch/2
  Switch/1 -> OutputK[x][y]/1
  OutputJ[x][y]/1 -> Switch1/3, Min1/1, Relational Operator2/2, Product/1, Switch/3
  Constant1/1 -> Relational Operator1/1
  Relational Operator1/1 -> Switch1/2
  Switch1/1 -> Switch/1, Product1/1
  Switch2/1 -> OutputL[x][y]/1
  Constant6/1 -> Product/2  "ConstantI"
  Product/1 -> Abs/1
  Abs/1 -> Bias/1
  Bias/1 -> Divide/1
  Constant2/1 -> Divide/2
  Subtract/1 -> Max/1
  Constant3/1 -> Max/2
  Constant5/1 -> Product1/2  "ConstantC"
  Product1/1 -> Abs1/1
  Abs1/1 -> Subtract/2
  Constant4/1 -> Relational Operator2/1
  Relational Operator2/1 -> Switch3/2
  Switch3/1 -> Switch2/1
  Divide/1 -> Switch3/3, Switch2/3
  Max/1 -> Switch3/1
  OutputKOld[x][y]/1 -> Delay/1
  OutputLOld[x][y]/1 -> Delay1/1
  Delay1/1 -> Subtract/1, Relational Operator1/2
  Min1/1 -> Switch1/1
  Delay/1 -> Min1/2

== system Simulink_Model/Subsystem/Requirement9/ComputeOutputM[0] ==
  OutputE[x][0] : Inport
  OutputE[x][1] : Inport  Port=2
  Add Constant : Bias  Bias=1
  Add Constant1 : Bias  Bias=-1
  Compare To Constant : simulink/Logic and Bit Operations/Compare To Constant  relop=>=  const=0  OutDataTypeStr=boolean
  Constant : Constant  Value=2
  Divide : Product  Inputs=*/
  Sum : Sum  Inputs=|++
  Switch : Switch  Criteria=u2 > Threshold
  OutputM[x] : Outport
  wires:
  OutputE[x][0]/1 -> Sum/1
  OutputE[x][1]/1 -> Sum/2
  Sum/1 -> Add Constant1/1, Add Constant/1, Compare To Constant/1
  Compare To Constant/1 -> Switch/2
  Add Constant/1 -> Switch/1
  Add Constant1/1 -> Switch/3
  Divide/1 -> OutputM[x]/1
  Switch/1 -> Divide/1
  Constant/1 -> Divide/2

== system Simulink_Model/Subsystem/Requirement9/ComputeOutputM[0]1 ==
  OutputE[x][0] : Inport
  OutputE[x][1] : Inport  Port=2
  Add Constant : Bias  Bias=1
  Add Constant1 : Bias  Bias=-1
  Compare To Constant : simulink/Logic and Bit Operations/Compare To Constant  relop=>=  const=0  OutDataTypeStr=boolean
  Constant : Constant  Value=2
  Divide : Product  Inputs=*/
  Sum : Sum  Inputs=|++
  Switch : Switch  Criteria=u2 > Threshold
  OutputM[x] : Outport
  wires:
  OutputE[x][0]/1 -> Sum/1
  OutputE[x][1]/1 -> Sum/2
  Sum/1 -> Add Constant1/1, Add Constant/1, Compare To Constant/1
  Compare To Constant/1 -> Switch/2
  Add Constant/1 -> Switch/1
  Add Constant1/1 -> Switch/3
  Divide/1 -> OutputM[x]/1
  Switch/1 -> Divide/1
  Constant/1 -> Divide/2

== system Simulink_Model/Subsystem/Verification2/ComputeStateB[0] ==
  OutputB[x][0] : Inport
  OutputB[x][1] : Inport  Port=2
  Abs : Abs
  Add : Sum
  Constant : Constant  Value=0
  Constant1 : Constant  Value=2
  Constant2 : Constant  Value=0
  Constant4 : Constant  Value=ConstantJ
  Delay : Delay  DelayLength=1  InitialCondition=0
  Minus : Sum  Inputs=+-
  Relational Operator : RelationalOperator  Operator=~=  OutDataTypeStr=boolean  RndMeth=Simplest
  Relational Operator1 : RelationalOperator  Operator=<=  OutDataTypeStr=boolean  RndMeth=Simplest
  Subsystem Reference : Subsystem  ReferencedSubsystem=ComputeState
  Switch : Switch  Criteria=u2 > Threshold
  Switch1 : Switch  Criteria=u2 > Threshold
  StateB[x] : Outport
  wires:
  OutputB[x][0]/1 -> Minus/1, Relational Operator/1
  OutputB[x][1]/1 -> Relational Operator/2, Minus/2
  Constant/1 -> Switch/1
  Constant1/1 -> Switch/3
  Subsystem Reference/1 -> StateB[x]/1
  Switch/1 -> Subsystem Reference/1
  Relational Operator/1 -> Switch1/2
  Switch1/1 -> Delay/1, Relational Operator1/1
  Minus/1 -> Abs/1
  Abs/1 -> Add/1
  Delay/1 -> Add/2
  Add/1 -> Switch1/1
  Constant2/1 -> Switch1/3
  Relational Operator1/1 -> Switch/2
  Constant4/1 -> Relational Operator1/2  "ConstantJ"

== system Simulink_Model/Subsystem/Verification2/ComputeStateB[1] ==
  OutputB[x][0] : Inport
  OutputB[x][1] : Inport  Port=2
  Abs : Abs
  Add : Sum
  Constant : Constant  Value=0
  Constant1 : Constant  Value=2
  Constant2 : Constant  Value=0
  Constant4 : Constant  Value=ConstantJ
  Delay : Delay  DelayLength=1  InitialCondition=0
  Minus : Sum  Inputs=+-
  Relational Operator : RelationalOperator  Operator===  OutDataTypeStr=boolean  RndMeth=Simplest
  Relational Operator1 : RelationalOperator  Operator=<=  OutDataTypeStr=boolean  RndMeth=Simplest
  Subsystem Reference : Subsystem  ReferencedSubsystem=ComputeState
  Switch : Switch  Criteria=u2 > Threshold
  Switch1 : Switch  Criteria=u2 > Threshold
  StateB[x] : Outport
  wires:
  OutputB[x][0]/1 -> Minus/1, Relational Operator/1
  OutputB[x][1]/1 -> Relational Operator/2, Minus/2
  Constant/1 -> Switch/1
  Constant1/1 -> Switch/3
  Subsystem Reference/1 -> StateB[x]/1
  Switch/1 -> Subsystem Reference/1
  Relational Operator/1 -> Switch1/2
  Switch1/1 -> Delay/1, Relational Operator1/1
  Minus/1 -> Abs/1
  Abs/1 -> Add/1
  Delay/1 -> Add/2
  Add/1 -> Switch1/1
  Constant2/1 -> Switch1/3
  Relational Operator1/1 -> Switch/2
  Constant4/1 -> Relational Operator1/2  "ConstantJ"

== system Simulink_Model/Subsystem/Verification4/ComputeStateD[0] ==
  OutputP[x] : Inport
  Constant : Constant  Value=2
  Constant1 : Constant  Value=0
  Constant4 : Constant  Value=ConstantK
  Relational Operator : RelationalOperator  Operator=<=  OutDataTypeStr=boolean  RndMeth=Simplest
  Subsystem Reference : Subsystem  ReferencedSubsystem=ComputeState
  Switch : Switch  Criteria=u2 > Threshold
  StateD[X] : Outport
  wires:
  Subsystem Reference/1 -> StateD[X]/1
  OutputP[x]/1 -> Relational Operator/1
  Constant4/1 -> Relational Operator/2  "ConstantK"
  Relational Operator/1 -> Switch/2
  Switch/1 -> Subsystem Reference/1
  Constant/1 -> Switch/3
  Constant1/1 -> Switch/1

== system Simulink_Model/Subsystem/Verification4/ComputeStateD[1] ==
  OutputP[x] : Inport
  Constant : Constant  Value=2
  Constant1 : Constant  Value=0
  Constant4 : Constant  Value=ConstantK
  Relational Operator : RelationalOperator  Operator=<=  OutDataTypeStr=boolean  RndMeth=Simplest
  Subsystem Reference : Subsystem  ReferencedSubsystem=ComputeState
  Switch : Switch  Criteria=u2 > Threshold
  StateD[X] : Outport
  wires:
  Subsystem Reference/1 -> StateD[X]/1
  OutputP[x]/1 -> Relational Operator/1
  Constant4/1 -> Relational Operator/2  "ConstantK"
  Relational Operator/1 -> Switch/2
  Switch/1 -> Subsystem Reference/1
  Constant/1 -> Switch/3
  Constant1/1 -> Switch/1

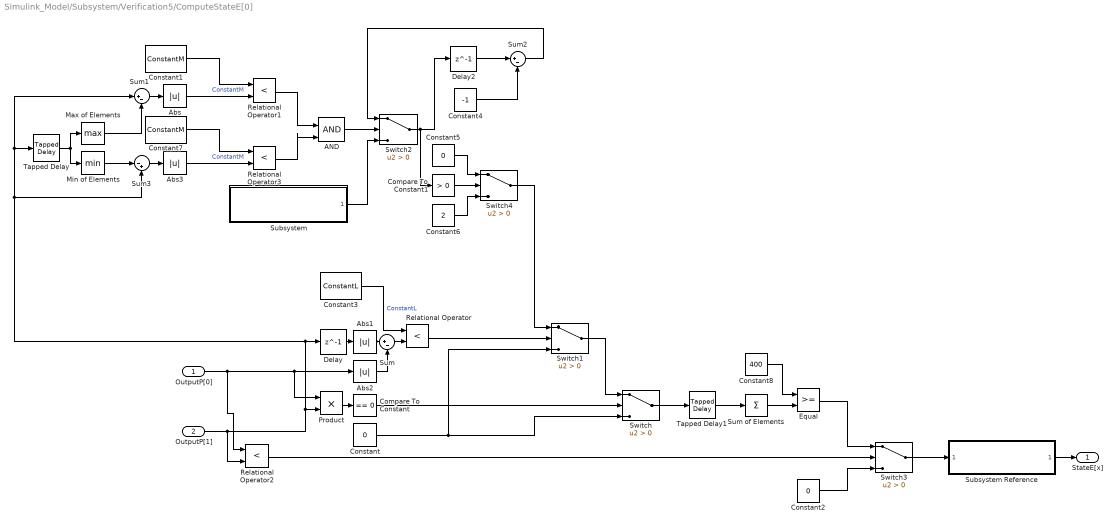
== system Simulink_Model/Subsystem/Verification5/ComputeStateE[0] ==
  OutputP[0] : Inport
  OutputP[1] : Inport  Port=2
  AND : Logic  IconShape=distinctive  AllPortsSameDT=off  OutDataTypeStr=boolean
  Abs{,1..3} (4 alike) : Abs
  Compare To Constant : simulink/Logic and Bit Operations/Compare To Constant  relop===  const=0  OutDataTypeStr=boolean
  Compare To Constant1 : simulink/Logic and Bit Operations/Compare To Constant  relop=>  const=0  OutDataTypeStr=boolean
  Constant : Constant  Value=0
  Constant1 : Constant  Value=ConstantM
  Constant2 : Constant  Value=0
  Constant3 : Constant  Value=ConstantL
  Constant4 : Constant  Value=-1
  Constant5 : Constant  Value=0
  Constant6 : Constant  Value=2
  Constant7 : Constant  Value=ConstantM
  Constant8 : Constant  Value=400
  Delay : Delay  DelayLength=1  InitialCondition=0
  Delay2 : Delay  DelayLength=1  InitialCondition=0
  Equal : RelationalOperator  OutDataTypeStr=boolean  RndMeth=Simplest
  Max of Elements : MinMax  Function=max
  Min of Elements : MinMax
  Product : Product
  Relational Operator{,1..3} (4 alike) : RelationalOperator  Operator=<  OutDataTypeStr=boolean  RndMeth=Simplest
  Subsystem : Subsystem  ReferencedSubsystem=CyclesFromSeconds  sec=30
  Subsystem Reference : Subsystem  ReferencedSubsystem=ComputeState
  Sum : Sum  Inputs=|+-
  Sum of Elements : Sum  Inputs=+
  Sum1 : Sum  Inputs=|+-
  Sum2 : Sum  Inputs=|+-
  Sum3 : Sum  Inputs=|-+
  Switch{,1..4} (5 alike) : Switch  Criteria=u2 > Threshold
  Tapped Delay : simulink/Discrete/Tapped Delay  vinit=0.0  samptime=-1  NumDelays=200  DelayOrder=Oldest  includeCurrent=off
  Tapped Delay1 : simulink/Discrete/Tapped Delay  vinit=0.0  samptime=-1  NumDelays=200  DelayOrder=Oldest  includeCurrent=off
  StateE[x] : Outport
  wires:
  OutputP[0]/1 -> Relational Operator2/1, Product/1, Abs2/1
  OutputP[1]/1 -> Relational Operator2/2, Sum3/2, Tapped Delay/1, Sum1/1, Delay/1, Product/2
  Constant/1 -> Switch1/3, Switch/3
  Product/1 -> Compare To Constant/1
  Compare To Constant/1 -> Switch/2
  Constant3/1 -> Relational Operator/1  "ConstantL"
  Sum/1 -> Relational Operator/2
  Relational Operator/1 -> Switch1/2
  Switch1/1 -> Switch/1
  Subsystem Reference/1 -> StateE[x]/1
  Relational Operator2/1 -> Switch3/2
  Constant2/1 -> Switch3/3
  Switch3/1 -> Subsystem Reference/1
  Sum1/1 -> Abs/1
  Abs/1 -> Relational Operator1/2
  Constant1/1 -> Relational Operator1/1  "ConstantM"
  Switch2/1 -> Compare To Constant1/1, Delay2/1
  Delay2/1 -> Sum2/1
  Subsystem/1 -> Switch2/3
  Constant4/1 -> Sum2/2
  Sum2/1 -> Switch2/1
  Compare To Constant1/1 -> Switch4/2
  Constant5/1 -> Switch4/1
  Constant6/1 -> Switch4/3
  Switch4/1 -> Switch1/1
  Delay/1 -> Abs1/1
  Abs1/1 -> Sum/1
  Abs2/1 -> Sum/2
  Tapped Delay/1 -> Min of Elements/1, Max of Elements/1
  Max of Elements/1 -> Sum1/2
  Min of Elements/1 -> Sum3/1
  Sum3/1 -> Abs3/1
  Abs3/1 -> Relational Operator3/2
  Constant7/1 -> Relational Operator3/1  "ConstantM"
  AND/1 -> Switch2/2
  Relational Operator1/1 -> AND/1
  Relational Operator3/1 -> AND/2
  Switch/1 -> Tapped Delay1/1
  Tapped Delay1/1 -> Sum of Elements/1
  Constant8/1 -> Equal/1
  Equal/1 -> Switch3/1
  Sum of Elements/1 -> Equal/2
